simulink model "Assignment1_735_Simulink_Ver3"  (R2022a)
settings: Solver=VariableStepAuto  StartTime=0.0  StopTime=8  RelTol=1e-3
model workspace (MAT data in the model file):
  Vdc = 1
undefined symbols (not defined in the file or in its folder): Ion, Lithium
libraries: spsSeriesRLCBranchLib x8, spsIGBTDiodeLib x6, spsBreakerLib x4, spsVoltageMeasurementLib x3, slpidlib x2, spsCurrentMeasurementLib x2, spsTHDLib x2, spsBatteryLib x1, eePwmGenerator x1, plecslib_extras2 x1, spspowerguiLib x1
settings Model: Creator=giaco  LastModifiedBy=maxje
settings SolverCC: AlgebraicLoopSolver=TrustRegion
settings DebuggingCC: UnconnectedInputMsg=warning  UnconnectedOutputMsg=warning  UnconnectedLineMsg=warning  SFMachineParentedDataDiag=warning

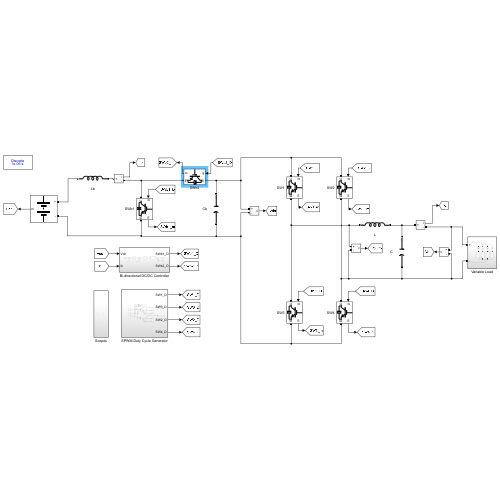
[thumbnail: Simulink's stored preview of the top-level diagram]
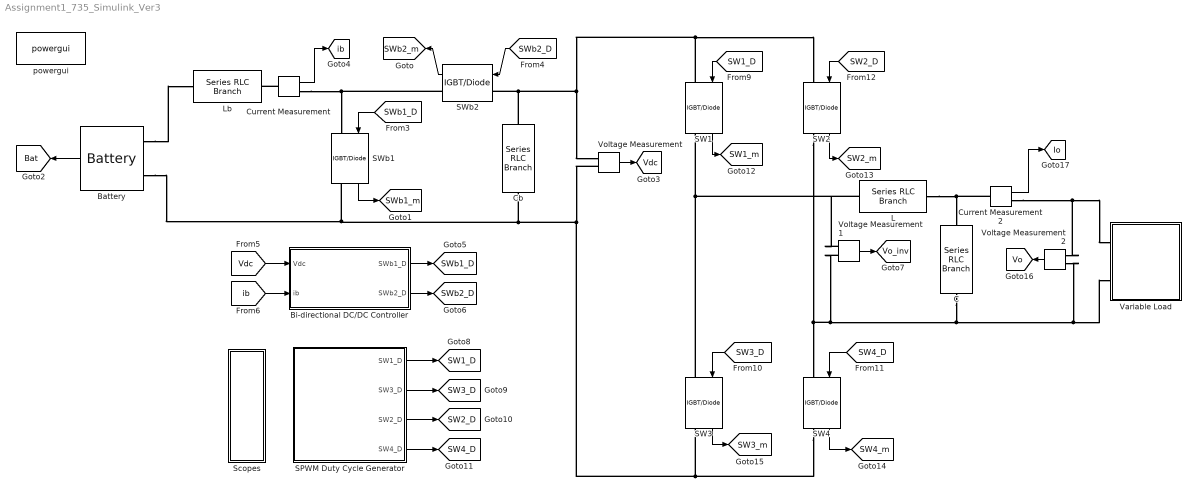
== system Assignment1_735_Simulink_Ver3 ==
  Battery : spsBatteryLib/Battery  BatType=Lithium-Ion  ShowTempParam=off  ThermalPreset=no  ShowAgeParam=off  NomV=24  NomQ=6.5  SOC=30  Batt_Tr=30  PresetModel=on  MaxQ=6.5  MinV=18  FullV=27.9357  Dis_rate=2.8261  R=0.036923  Normal_OP=5.8783  expZone="[25.9293     0.319348]"  current=[6.5 13 32.5]  Units=Time  Tci=20  NomT=20  T2=-30  MaxQ2=4.8  FullV2=7.1  Normal_OP2=5.655  expZone2="[6.58           1]"  Rca=0.6  ti=2000  Dp=0  Neq0=0  Tsim=1e6  Ta1=25  Qeol=5.4*0.9  Reol=0.013333*1.2  Char_age=[2.3478, 3]  Dis_age=[2.3478, 10]  N1=1500  N2=10500  N3=1000  N4=1400  Ta2=45  N5=950
  Bi-directional DC/DC Controller : Subsystem
  C : spsSeriesRLCBranchLib/Series RLC Branch  LConnTagsString=__new0  RConnTagsString=__new0  BranchType=C  Resistance=70.71  Inductance=1e-3  SetiL0=off  InitialCurrent=0  Capacitance=30e-6  Setx0=off  InitialVoltage=0  Measurements=None
  Cb : spsSeriesRLCBranchLib/Series RLC Branch  LConnTagsString=__new0  RConnTagsString=__new0  BranchType=C  Resistance=70.71  Inductance=1e-3  SetiL0=off  InitialCurrent=0  Capacitance=33e-3  Setx0=off  InitialVoltage=0  Measurements=None
  Current Measurement : spsCurrentMeasurementLib/Current Measurement  PhasorSimulation=off  OutputType=Complex  PSBequivalent=0
  Current Measurement2 : spsCurrentMeasurementLib/Current Measurement  PhasorSimulation=off  OutputType=Complex  PSBequivalent=0
  L : spsSeriesRLCBranchLib/Series RLC Branch  LConnTagsString=__new0  RConnTagsString=__new0  BranchType=L  Resistance=70.71  Inductance=880e-6  SetiL0=off  InitialCurrent=0  Capacitance=1e-6  Setx0=off  InitialVoltage=0  Measurements=None
  Lb : spsSeriesRLCBranchLib/Series RLC Branch  LConnTagsString=__new0  RConnTagsString=__new0  BranchType=L  Resistance=70.71  Inductance=1e-3  SetiL0=off  InitialCurrent=0  Capacitance=1e-6  Setx0=off  InitialVoltage=0  Measurements=None
  SPWM Duty Cycle Generator : Subsystem
  SW{1..4} (4 alike) : spsIGBTDiodeLib/IGBT//Diode  Ron=0.0047  Rs=1e5  Cs=inf  Measurements=on
  SWb1 : spsIGBTDiodeLib/IGBT//Diode  Ron=0.0047  Rs=1e5  Cs=inf  Measurements=on
  SWb2 : spsIGBTDiodeLib/IGBT//Diode  Ron=0.0047  Rs=1e5  Cs=inf  Measurements=on
  Scopes : Subsystem
  Variable Load : Subsystem
  Voltage Measurement : spsVoltageMeasurementLib/Voltage Measurement  PhasorSimulation=off  OutputType=Complex  PSBequivalent=0
  Voltage Measurement1 : spsVoltageMeasurementLib/Voltage Measurement  PhasorSimulation=off  OutputType=Complex  PSBequivalent=0
  Voltage Measurement2 : spsVoltageMeasurementLib/Voltage Measurement  PhasorSimulation=off  OutputType=Complex  PSBequivalent=0
  powergui : spspowerguiLib/powergui  Priority=1  SimulationMode=Discrete  SampleTime=1e-6  frequency=60  Iterations=50  frequencyindice=0  Pbase=100e6  ErrMax=1e-4  UnitsV=kV  UnitsW=MW  buscounter=0  FunctionMessages=off  echomessages=off  EnableUseOfTLC=off  CurrentSourceSwitches=off  DisableSnubberDevices=off  DisableRonSwitches=off  DisableVfSwitches=off  DisplayEquations=off  AutomaticDiscreteSolvers=off  SolverType=Tustin/Backward Euler (TBE)  Interpol=off  ExternalGateDelay=off  methode=off  Ts=100  x0status=blocks  SPID=on  SwTol=0  HookPort=off  NonlinearTolerance=1e-4  nMaxIteration=100  ContinueOnMaxIteration=off  RestoreLinks=warning  ResistiveCurrentMeasurement=off  Frange=[0:2:500]  Ylog=off  Xlog=on  ShowGrid=off  save=off  variable=ZData  structure=ScopeData  ZoomFFT=off  StartTime=0.0  cycles=1  DisplayStyle=1  fundamental=60  FreqAxis=off  MaxFrequency=1000  frequencyindicesteady=1  RmsSteady=1  display=off
  tag scope: Bat=global, Io=global, SW1_D=global, SW1_m=global, SW2_D=global, SW2_m=global, SW3_D=global, SW3_m=global, SW4_D=global, SW4_m=global, SWb1_D=global, SWb1_m=global, SWb2_D=global, SWb2_m=global, Vdc=global, Vo=global, Vo_inv=global, ib=global
  wires:
  SWb2/1 -> [SWb2_m]
  SWb1/1 -> [SWb1_m]
  Battery/1 -> [Bat]
  Voltage Measurement/1 -> [Vdc]
  Bi-directional DC/DC Controller/1(SWb1_D) -> [SWb1_D]
  Bi-directional DC/DC Controller/2(SWb2_D) -> [SWb2_D]
  Current Measurement/1 -> [ib]
  [SWb1_D] -> SWb1/1
  [SWb2_D] -> SWb2/1
  Voltage Measurement1/1 -> [Vo_inv]
  [SW1_D] -> SW1/1
  [SW3_D] -> SW3/1
  [SW2_D] -> SW2/1
  [SW4_D] -> SW4/1
  SPWM Duty Cycle Generator/1(SW1_D) -> [SW1_D]
  SPWM Duty Cycle Generator/2(SW3_D) -> [SW3_D]
  SPWM Duty Cycle Generator/3(SW2_D) -> [SW2_D]
  SPWM Duty Cycle Generator/4(SW4_D) -> [SW4_D]
  SW1/1 -> [SW1_m]
  SW2/1 -> [SW2_m]
  SW4/1 -> [SW4_m]
  SW3/1 -> [SW3_m]
  [Vdc] -> Bi-directional DC/DC Controller/1(Vdc)
  [ib] -> Bi-directional DC/DC Controller/2(ib)
  Voltage Measurement2/1 -> [Vo]
  Current Measurement2/1 -> [Io]
  connections:
  SWb2/RConn1 -- SWb1/LConn1 -- Current Measurement/RConn1
  Battery/LConn1 -- Lb/LConn1
  SW1/LConn1 -- Voltage Measurement/LConn1 -- Cb/LConn1 -- SWb2/LConn1 -- SW2/LConn1
  Current Measurement/LConn1 -- Lb/RConn1
  SW3/LConn1 -- SW1/RConn1 -- L/LConn1 -- Voltage Measurement1/LConn1
  L/RConn1 -- Current Measurement2/LConn1 -- C/LConn1
  Current Measurement2/RConn1 -- Voltage Measurement2/LConn1 -- Variable Load/LConn1
  SW4/RConn1 -- Voltage Measurement/LConn2 -- Cb/RConn1 -- Battery/LConn2 -- SWb1/RConn1 -- SW3/RConn1
  Voltage Measurement1/LConn2 -- SW2/RConn1 -- SW4/LConn1 -- Variable Load/LConn2 -- Voltage Measurement2/LConn2 -- C/RConn1

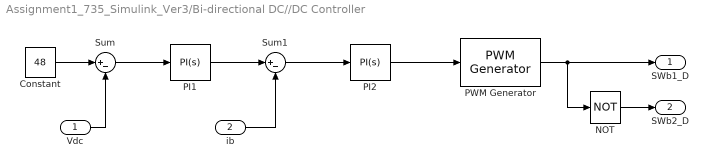
== system Assignment1_735_Simulink_Ver3/Bi-directional DC//DC Controller ==
  Vdc : Inport
  ib : Inport  Port=2
  Constant : Constant  Value=48
  NOT : Logic  Operator=NOT  IconShape=distinctive  AllPortsSameDT=off  OutDataTypeStr=boolean
  PI1 : slpidlib/PID Controller  Controller=PI  Form=Parallel  TimeDomain=Continuous-time  UseExternalTs=off  SampleTime=-1  IntegratorMethod=Forward Euler  FilterMethod=Forward Euler  ControllerParametersSource=internal  P=1.43117591255602  I=4.16218363897788  UseKiTs=off  D=0  N=100  UseFilter=on  TunerSelectOption=Transfer Function Based (PID Tuner App)  InitialConditionSource=internal  InitialConditionForIntegrator=0  InitialConditionForFilter=0  DifferentiatorICPrevScaledInput=0  ExternalReset=none  TrackingMode=off  Kt=1  LimitOutput=off  SatLimitsSource=internal  UpperSaturationLimit=inf  LowerSaturationLimit=-inf  LinearizeAsGain=on  AntiWindupMode=none  Kb=1  POutMin=[]  POutMax=[]  IOutMin=[]  IOutMax=[]  DOutMin=[]  DOutMax=[]  NOutMin=[]  NOutMax=[]  SumOutMin=[]  SumOutMax=[]  SaturationOutMin=[]  SaturationOutMax=[]  PParamMin=[]  PParamMax=[]  IParamMin=[]  IParamMax=[]  DParamMin=[]  DParamMax=[]  NParamMin=[]  NParamMax=[]  KbParamMin=[]  KbParamMax=[]  KtParamMin=[]  KtParamMax=[]  KbOutMin=[]  KbOutMax=[]  KtOutMin=[]  KtOutMax=[]  IntegratorOutMin=[]  IntegratorOutMax=[]  FilterOutMin=[]  FilterOutMax=[]  SumI1OutMin=[]  SumI1OutMax=[]  SumI2OutMin=[]  SumI2OutMax=[]  SumI3OutMin=[]  SumI3OutMax=[]  SumI4OutMin=[]  SumI4OutMax=[]  SumDOutMin=[]  SumDOutMax=[]  DifferentiatorOutMin=[]  DifferentiatorOutMax=[]  FilterDiffOutCoefMin=[]  FilterDiffOutCoefMax=[]  ReciprocalOutMin=[]  ReciprocalOutMax=[]  SumDenOutMin=[]  SumDenOutMax=[]  SumNumOutMin=[]  SumNumOutMax=[]  DivideOutMin=[]  DivideOutMax=[]  UdiffTsProdOutMin=[]  UdiffTsProdOutMax=[]  NTsProdOutMin=[]  NTsProdOutMax=[]  UintegralTsProdOutMin=[]  UintegralTsProdOutMax=[]  UngainTsProdOutMin=[]  UngainTsProdOutMax=[]  IntegratorContinuousStateAttributes=''  IntegratorStateMustResolveToSignalObject=off  IntegratorRTWStateStorageClass=Auto  FilterContinuousStateAttributes=''  FilterStateMustResolveToSignalObject=off  FilterRTWStateStorageClass=Auto  ParallelPVariant=InternalParameters  IdealPVariant=Disabled  IVariant=InternalParameters  DVariant=Disabled  IntegratorVariant=Continuous  SatVariant=Disabled  AWVariant=Passthrough  PCopyVariant=Disabled  TRVariant=Disabled  FdbkBlocksVariant=Forward  IdealPFdbkVariant=Disabled  SatFdbkVariant=Disabled  DerivativeFilterVariant=Disabled  NVariant=Disabled  NCopyVariant=Disabled_SignalSpec  FilterICVariant=Disabled  IntegratorICVariant=InternalICs  ExternalResetVariant=Disabled  TRSumVariant=Passthrough  SumFdbkVariant=Disabled  SumVariant=Sum_PI  TsampFilterVariant=InternalTs  TsampNgainVariant=Passthrough  TsampIntegralVariant=Passthrough  ExternalSaturationOutDataTypeStr=Inherit: Same as second input  aMode=0
  PI2 : slpidlib/PID Controller  Controller=PI  Form=Parallel  TimeDomain=Continuous-time  UseExternalTs=off  SampleTime=-1  IntegratorMethod=Forward Euler  FilterMethod=Forward Euler  ControllerParametersSource=internal  P=0.658922515700881  I=967.39616296182  UseKiTs=off  D=0  N=100  UseFilter=on  TunerSelectOption=Transfer Function Based (PID Tuner App)  InitialConditionSource=internal  InitialConditionForIntegrator=0  InitialConditionForFilter=0  DifferentiatorICPrevScaledInput=0  ExternalReset=none  TrackingMode=off  Kt=1  LimitOutput=off  SatLimitsSource=internal  UpperSaturationLimit=inf  LowerSaturationLimit=-inf  LinearizeAsGain=on  AntiWindupMode=none  Kb=1  POutMin=[]  POutMax=[]  IOutMin=[]  IOutMax=[]  DOutMin=[]  DOutMax=[]  NOutMin=[]  NOutMax=[]  SumOutMin=[]  SumOutMax=[]  SaturationOutMin=[]  SaturationOutMax=[]  PParamMin=[]  PParamMax=[]  IParamMin=[]  IParamMax=[]  DParamMin=[]  DParamMax=[]  NParamMin=[]  NParamMax=[]  KbParamMin=[]  KbParamMax=[]  KtParamMin=[]  KtParamMax=[]  KbOutMin=[]  KbOutMax=[]  KtOutMin=[]  KtOutMax=[]  IntegratorOutMin=[]  IntegratorOutMax=[]  FilterOutMin=[]  FilterOutMax=[]  SumI1OutMin=[]  SumI1OutMax=[]  SumI2OutMin=[]  SumI2OutMax=[]  SumI3OutMin=[]  SumI3OutMax=[]  SumI4OutMin=[]  SumI4OutMax=[]  SumDOutMin=[]  SumDOutMax=[]  DifferentiatorOutMin=[]  DifferentiatorOutMax=[]  FilterDiffOutCoefMin=[]  FilterDiffOutCoefMax=[]  ReciprocalOutMin=[]  ReciprocalOutMax=[]  SumDenOutMin=[]  SumDenOutMax=[]  SumNumOutMin=[]  SumNumOutMax=[]  DivideOutMin=[]  DivideOutMax=[]  UdiffTsProdOutMin=[]  UdiffTsProdOutMax=[]  NTsProdOutMin=[]  NTsProdOutMax=[]  UintegralTsProdOutMin=[]  UintegralTsProdOutMax=[]  UngainTsProdOutMin=[]  UngainTsProdOutMax=[]  IntegratorContinuousStateAttributes=''  IntegratorStateMustResolveToSignalObject=off  IntegratorRTWStateStorageClass=Auto  FilterContinuousStateAttributes=''  FilterStateMustResolveToSignalObject=off  FilterRTWStateStorageClass=Auto  ParallelPVariant=InternalParameters  IdealPVariant=Disabled  IVariant=InternalParameters  DVariant=Disabled  IntegratorVariant=Continuous  SatVariant=Disabled  AWVariant=Passthrough  PCopyVariant=Disabled  TRVariant=Disabled  FdbkBlocksVariant=Forward  IdealPFdbkVariant=Disabled  SatFdbkVariant=Disabled  DerivativeFilterVariant=Disabled  NVariant=Disabled  NCopyVariant=Disabled_SignalSpec  FilterICVariant=Disabled  IntegratorICVariant=InternalICs  ExternalResetVariant=Disabled  TRSumVariant=Passthrough  SumFdbkVariant=Disabled  SumVariant=Sum_PI  TsampFilterVariant=InternalTs  TsampNgainVariant=Passthrough  TsampIntegralVariant=Passthrough  ExternalSaturationOutDataTypeStr=Inherit: Same as second input  aMode=0
  PWM Generator : eePwmGenerator/PWM Generator  CarrCount=Up  Tper=0.000125  Tdelay=0  Ts=1.25e-5
  Sum : Sum  Inputs=|+-
  Sum1 : Sum  Inputs=|+-
  SWb1_D : Outport
  SWb2_D : Outport  Port=2
  wires:
  Sum/1 -> PI1/1
  PWM Generator/1 -> NOT/1, SWb1_D/1
  Constant/1 -> Sum/1
  NOT/1 -> SWb2_D/1
  Vdc/1 -> Sum/2
  ib/1 -> Sum1/2
  PI2/1 -> PWM Generator/1
  Sum1/1 -> PI2/1
  PI1/1 -> Sum1/1

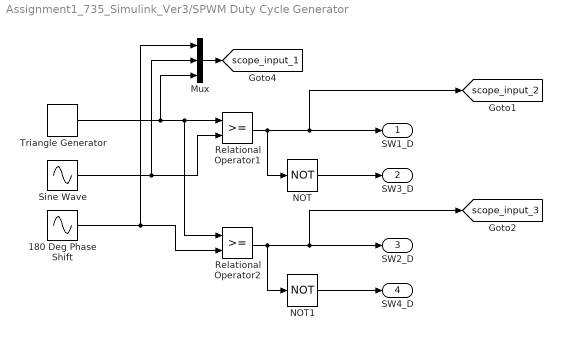
== system Assignment1_735_Simulink_Ver3/SPWM Duty Cycle Generator ==
  180 Deg Phase Shift : Sin  Amplitude=0.95  Frequency=2*pi*50  Phase=pi  SampleTime=0
  Mux : Mux  Inputs=3
  NOT : Logic  Operator=NOT  IconShape=distinctive  AllPortsSameDT=off  OutDataTypeStr=boolean
  NOT1 : Logic  Operator=NOT  IconShape=distinctive  AllPortsSameDT=off  OutDataTypeStr=boolean
  Relational Operator1 : RelationalOperator  OutDataTypeStr=boolean  RndMeth=Simplest  InputSameDT=off
  Relational Operator2 : RelationalOperator  OutDataTypeStr=boolean  RndMeth=Simplest  InputSameDT=off
  Sine Wave : Sin  Amplitude=0.95  Frequency=2*pi*50  SampleTime=0
  Triangle Generator : plecslib_extras2/Modulators/Triangle Generator  fc=8050  offset=0  range=[-1 1]
      settings: SourceProductName=PLECS Extras
  SW1_D : Outport
  SW3_D : Outport  Port=2
  SW2_D : Outport  Port=3
  SW4_D : Outport  Port=4
  tag scope: scope_input_1=global, scope_input_2=global, scope_input_3=global
  wires:
  Triangle Generator/1 -> Mux/3, Relational Operator1/1, Relational Operator2/1
  Relational Operator1/1 -> [scope_input_2], SW1_D/1, NOT/1
  NOT1/1 -> SW4_D/1
  Relational Operator2/1 -> [scope_input_3], SW2_D/1, NOT1/1
  180 Deg Phase Shift/1 -> Mux/1, Relational Operator2/2
  NOT/1 -> SW3_D/1
  Mux/1 -> [scope_input_1]
  Sine Wave/1 -> Mux/2, Relational Operator1/2

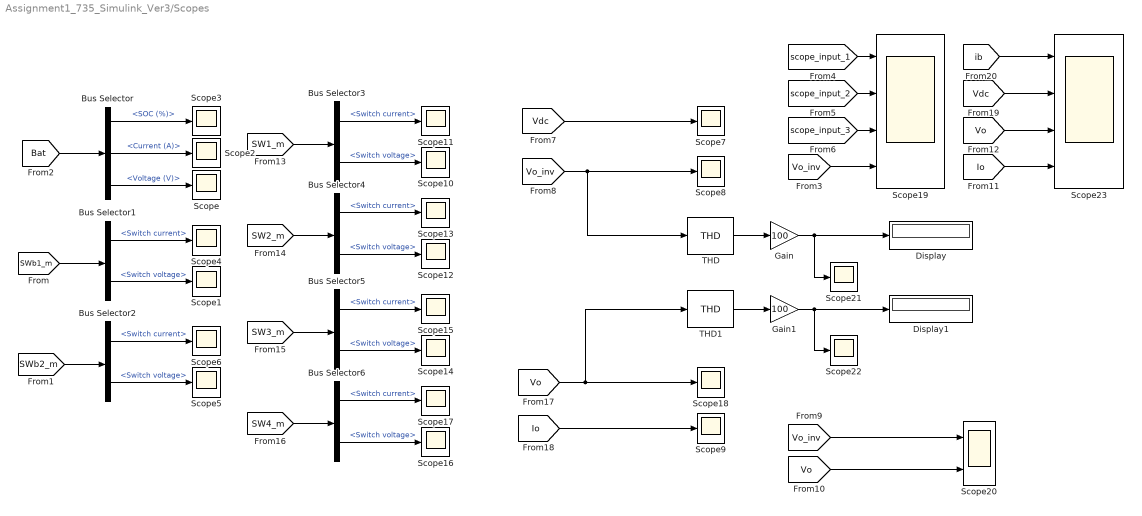
== system Assignment1_735_Simulink_Ver3/Scopes ==
  Bus Selector : BusSelector  OutputSignals=SOC (%),Current (A),Voltage (V)
  Bus Selector{1..6} (6 alike) : BusSelector  OutputSignals=Switch current,Switch voltage
  Display : Display
  Display1 : Display
  Gain : Gain  Gain=100
  Gain1 : Gain  Gain=100
  Scope{,1..18,21..22} (21 alike) : Scope
  Scope19 : Scope  NumInputPorts=4
  Scope20 : Scope  NumInputPorts=2
  Scope23 : Scope  NumInputPorts=4
  THD : spsTHDLib/THD  Freq=50  Ts=0
      settings: SourceProductBaseCode=PS
  THD1 : spsTHDLib/THD  Freq=50  Ts=0
      settings: SourceProductBaseCode=PS
  wires:
  Bus Selector1/2 -> Scope1/1  "<Switch voltage>"
  [SW1_m] -> Bus Selector3/1
  [Vo] -> Scope18/1, THD1/1
  Gain/1 -> Display/1, Scope21/1
  Bus Selector4/1 -> Scope13/1  "<Switch current>"
  [SWb1_m] -> Bus Selector1/1
  Bus Selector6/1 -> Scope17/1  "<Switch current>"
  Bus Selector/2 -> Scope2/1  "<Current (A)>"
  Bus Selector6/2 -> Scope16/1  "<Switch voltage>"
  [Vo_inv] -> Scope8/1, THD/1
  [Bat] -> Bus Selector/1
  Bus Selector1/1 -> Scope4/1  "<Switch current>"
  Gain1/1 -> Display1/1, Scope22/1
  Bus Selector2/2 -> Scope5/1  "<Switch voltage>"
  Bus Selector2/1 -> Scope6/1  "<Switch current>"
  Bus Selector3/2 -> Scope10/1  "<Switch voltage>"
  THD1/1 -> Gain1/1
  Bus Selector5/1 -> Scope15/1  "<Switch current>"
  [Vdc] -> Scope7/1
  Bus Selector3/1 -> Scope11/1  "<Switch current>"
  [SW2_m] -> Bus Selector4/1
  THD/1 -> Gain/1
  [SW3_m] -> Bus Selector5/1
  Bus Selector5/2 -> Scope14/1  "<Switch voltage>"
  Bus Selector4/2 -> Scope12/1  "<Switch voltage>"
  Bus Selector/1 -> Scope3/1  "<SOC (%)>"
  [SW4_m] -> Bus Selector6/1
  [SWb2_m] -> Bus Selector2/1
  Bus Selector/3 -> Scope/1  "<Voltage (V)>"
  [Io] -> Scope9/1
  [Vo_inv] -> Scope19/4
  [scope_input_1] -> Scope19/1
  [scope_input_2] -> Scope19/2
  [scope_input_3] -> Scope19/3
  [Vo_inv] -> Scope20/1
  [Vo] -> Scope20/2
  [Vo] -> Scope23/3
  [Io] -> Scope23/4
  [Vdc] -> Scope23/2
  [ib] -> Scope23/1

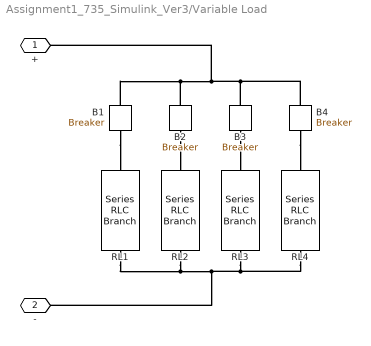
== system Assignment1_735_Simulink_Ver3/Variable Load ==
  B1 : spsBreakerLib/Breaker  InitialState=1  SwitchingTimes=[2]  External=off  BreakerResistance=0.01  SnubberResistance=1e6  SnubberCapacitance=inf  Measurements=None  MoreParameters=on  NoBreakLoop=off
      settings: SourceProductBaseCode=PS
  B2 : spsBreakerLib/Breaker  InitialState=0  SwitchingTimes=[2 4]  External=off  BreakerResistance=0.01  SnubberResistance=1e6  SnubberCapacitance=inf  Measurements=None  MoreParameters=on  NoBreakLoop=off
      settings: SourceProductBaseCode=PS
  B3 : spsBreakerLib/Breaker  InitialState=0  SwitchingTimes=[4 6]  External=off  BreakerResistance=0.01  SnubberResistance=1e6  SnubberCapacitance=inf  Measurements=None  MoreParameters=on  NoBreakLoop=off
      settings: SourceProductBaseCode=PS
  B4 : spsBreakerLib/Breaker  InitialState=0  SwitchingTimes=[6 8]  External=off  BreakerResistance=0.01  SnubberResistance=1e6  SnubberCapacitance=inf  Measurements=None  MoreParameters=on  NoBreakLoop=off
      settings: SourceProductBaseCode=PS
  RL1 : spsSeriesRLCBranchLib/Series RLC Branch  LConnTagsString=__new0  RConnTagsString=__new0  BranchType=R  Resistance=50  Inductance=1e-3  SetiL0=off  InitialCurrent=0  Capacitance=1e-3  Setx0=off  InitialVoltage=0  Measurements=None
  RL2 : spsSeriesRLCBranchLib/Series RLC Branch  LConnTagsString=__new0  RConnTagsString=__new0  BranchType=R  Resistance=100  Inductance=1e-3  SetiL0=off  InitialCurrent=0  Capacitance=1e-3  Setx0=off  InitialVoltage=0  Measurements=None
  RL3 : spsSeriesRLCBranchLib/Series RLC Branch  LConnTagsString=__new0  RConnTagsString=__new0  BranchType=R  Resistance=40  Inductance=1e-3  SetiL0=off  InitialCurrent=0  Capacitance=1e-3  Setx0=off  InitialVoltage=0  Measurements=None
  RL4 : spsSeriesRLCBranchLib/Series RLC Branch  LConnTagsString=__new0  RConnTagsString=__new0  BranchType=R  Resistance=80  Inductance=1e-3  SetiL0=off  InitialCurrent=0  Capacitance=1e-3  Setx0=off  InitialVoltage=0  Measurements=None
  + : PMIOPort  Side=Left
  - : PMIOPort  Port=2  Side=Left
  connections:
  RL1/RConn1 -- -/RConn1 -- RL4/RConn1 -- RL3/RConn1 -- RL2/RConn1
  B1/RConn1 -- RL1/LConn1
  B2/RConn1 -- RL2/LConn1
  B2/LConn1 -- B1/LConn1 -- B4/LConn1 -- B3/LConn1 -- +/RConn1
  B3/RConn1 -- RL3/LConn1
  B4/RConn1 -- RL4/LConn1
